simulink model "Boeing787_NewMission_ElectricalThermal_2013"  (R2013a)
settings: Solver=ode23tb  SolverMode=SingleTasking  StartTime=0.0  StopTime=18000  RelTol=1e-3
InitFcn:
  | load('SampleOutput.mat')
  | 
  | load('SampleFuelBurn.mat')
StartFcn:
  | tic
StopFcn:
  | ttt = toc
  | tend = eval(get_param(bdroot,'StopTime'));
  | disp(['Total Simulation Time (s) = ' num2str(ttt) 's']);
  | RTR =  ttt/tend
  | disp(['Simulation Speed is ' num2str(tend/ttt) 'x faster than real-time']);
values from neighbouring files (symbols this model uses):
  CurrentMission = Mission(i)    [mission_plan.m]
  seed = 1    [mission_plan.m]
undefined symbols (not defined in the file or in its folder): FuelBurn
libraries: PowerFlowLib x17, simulink x12, powerlib_meascontrol x1
(part 13 of 17)

== system Boeing787_NewMission_ElectricalThermal_2013/Electrical/230 Vac Distr ==
  note: Generator Bus 1
  note: Generator Bus 2
  Gen 1 : Inport
  Gen 2 : Inport  Port=2
  Gen 3 : Inport  Port=3
  Gen 4 : Inport  Port=4
  Gen 5 : Inport  Port=5
  Gen 6 : Inport  Port=6
  I_Bus : Inport  Port=7
  Gain : Gain  Gain=0.45
  Gain1 : Gain  Gain=0.55
  Gen Bus w/ APU switch : PowerFlowLib/Energy & Power Systems/Electrical/Systems/Gen Bus w// APU switch  LOWVLIMIT=90  UPVLIMIT=250  bus_st=2
  Gen Bus w/ APU switch1 : PowerFlowLib/Energy & Power Systems/Electrical/Systems/Gen Bus w// APU switch  LOWVLIMIT=90  UPVLIMIT=250  bus_st=2
  Terminator : Terminator
  Terminator1 : Terminator
  Vbus1 : Outport
  Vbus2 : Outport  Port=2
  tag scope: i_APU1=global, i_APU2=global, i_GND1=global, i_GND2=global, i_MAIN1=global, i_MAIN2=global
  wires:
  Gen Bus w/ APU switch/3 -> [i_APU1]
  Gen Bus w/ APU switch/4 -> [i_GND1]
  [Gen_Bus1] -> Gen Bus w/ APU switch/1
  Gen Bus w/ APU switch/2 -> [i_MAIN1]
  Gen Bus w/ APU switch1/3 -> [i_APU2]
  Gen Bus w/ APU switch1/4 -> [i_GND2]
  Gen Bus w/ APU switch1/2 -> [i_MAIN2]
  [Gen_Bus2] -> Gen Bus w/ APU switch1/1
  Gen 1/1 -> Gen Bus w/ APU switch/2
  Gen 3/1 -> Gen Bus w/ APU switch1/2
  Gen 5/1 -> Gen Bus w/ APU switch/3
  Gen 6/1 -> Gen Bus w/ APU switch1/3
  Gen Bus w/ APU switch/1 -> Vbus1/1
  Gen Bus w/ APU switch1/1 -> Vbus2/1
  I_Bus/1 -> Gain1/1, Gain/1
  Gain/1 -> Gen Bus w/ APU switch/6
  Gen 2/1 -> Terminator/1
  Gen 4/1 -> Terminator1/1
  Gain1/1 -> Gen Bus w/ APU switch1/6

== system Boeing787_NewMission_ElectricalThermal_2013/Electrical/Auto Transformer ==
  vqd0 : Inport
  iAC : Inport  Port=2
  Constant : Constant
  Constant1 : Constant  Value=115
  Control : Subsystem
  Saturation : Saturate  UpperLimit=20  LowerLimit=0
  Sum1 : Sum  Inputs=|++
  Transformer1 : Subsystem  AncestorBlock=PowerFlowLib/Energy & Power Systems/Electrical/Machines/Transformer  mask(Transformer){Rp=0.005, Rs=0.1, N1=400, N2=200}
      mask prompts: Rp "Primary Winding Resistance"; Rs "Secondary Winding Resistance"; N1 "Number of Turns in Primary"; N2 "Number of Turns in Secondary"
      mask help:
      | The user inputs and outputs are given below. Inputs to the model are:
      |
      | Block Inputs
      | #1: Primary voltage input [V]
      | #2: Secondary current input [A]
      |
      | Block Outputs
      | #1: Secondary voltage output [V]
      | #2: Primary current input [A]
      mask Help: eval('open(''Transformer Help.html'')');
      mask Display:
      | image(imread('Transformer.png'))
      | 
      | port_label('input',1,'{\bf V_i_n}','TexMode','on')
      | port_label('input',2,'{\bf I_o_u_t}','TexMode','on')
      | port_label('input',3,'{\bf u}','TexMode','on')
      | 
      | port_label('output',1,'{\bf V_o_u_t}','TexMode','on')
      | port_label('output',2,'{\bf I_i_n}','TexMode','on')
  vout : Outport
  iqd0 : Outport  Port=2
  wires:
  vqd0/1 -> Transformer1/1(Vin)
  Transformer1/2(Iin) -> iqd0/1
  iAC/1 -> Transformer1/2(Iout)
  Transformer1/1(Vout) -> Control/1(Vout), vout/1
  Sum1/1 -> Saturation/1
  Constant/1 -> Sum1/1
  Constant1/1 -> Control/2(ref)
  Saturation/1 -> Transformer1/3(u)
  Control/1(u) -> Sum1/2

== system Boeing787_NewMission_ElectricalThermal_2013/Electrical/Bus Controls ==
  Constant{1..5} (5 alike) : Constant
  Gen_Bus1 : Outport
  Gen_Bus2 : Outport  Port=2
  270V_DC_Bus : Outport  Port=3
  115V_AC_Bus : Outport  Port=4
  28V_DC_Bus : Outport  Port=5
  wires:
  Constant3/1 -> 28V_DC_Bus/1
  Constant5/1 -> 115V_AC_Bus/1
  Constant2/1 -> 270V_DC_Bus/1
  Constant4/1 -> Gen_Bus2/1
  Constant1/1 -> Gen_Bus1/1

== system Boeing787_NewMission_ElectricalThermal_2013/Electrical/DC Bus 1 ==
  Select : Inport
  VDC_1 : Inport  Port=2
  VDC_2 : Inport  Port=3
  Load current : Inport  Port=4
  Compare To Constant : simulink/Logic and Bit Operations/Compare To Constant  relop=<=  const=3.0  OutDataTypeStr=boolean
  Compare To Constant1 : simulink/Logic and Bit Operations/Compare To Constant  relop=<=  const=3.0  OutDataTypeStr=boolean
  Constant : Constant  Value=[0]
  Multiport Switch : MultiPortSwitch  Inputs=2
  Sum of Elements1 : Sum  Inputs=+
  Switch : Switch  Criteria=u2 ~= 0
  Switch1 : Switch  Criteria=u2 ~= 0
  Vbus : Outport
  IDC_1 : Outport  Port=2
  IDC_2 : Outport  Port=3
  wires:
  Load current/1 -> Sum of Elements1/1
  Multiport Switch/1 -> Vbus/1
  VDC_1/1 -> Multiport Switch/2
  VDC_2/1 -> Multiport Switch/3
  Select/1 -> Multiport Switch/1, Compare To Constant/1, Compare To Constant1/1
  Compare To Constant/1 -> Switch/2
  Compare To Constant1/1 -> Switch1/2
  Constant/1 -> Switch/3, Switch1/3
  Switch/1 -> IDC_1/1
  Switch1/1 -> IDC_2/1
  Sum of Elements1/1 -> Switch1/1, Switch/1

== system Boeing787_NewMission_ElectricalThermal_2013/Electrical/DC Bus 3 ==
  Select : Inport
  VDC_1 : Inport  Port=2
  VDC_2 : Inport  Port=3
  Load current : Inport  Port=4
  Compare To Constant : simulink/Logic and Bit Operations/Compare To Constant  relop=<=  const=3.0  OutDataTypeStr=boolean
  Compare To Constant1 : simulink/Logic and Bit Operations/Compare To Constant  relop=<=  const=3.0  OutDataTypeStr=boolean
  Constant : Constant  Value=[0]
  Multiport Switch : MultiPortSwitch  Inputs=2
  Sum of Elements : Sum  Inputs=+
  Switch : Switch  Criteria=u2 ~= 0
  Switch1 : Switch  Criteria=u2 ~= 0
  Vbus : Outport
  IDC_1 : Outport  Port=2
  IDC_2 : Outport  Port=3
  wires:
  Load current/1 -> Sum of Elements/1
  Multiport Switch/1 -> Vbus/1
  VDC_1/1 -> Multiport Switch/2
  VDC_2/1 -> Multiport Switch/3
  Select/1 -> Multiport Switch/1, Compare To Constant1/1, Compare To Constant/1
  Compare To Constant/1 -> Switch/2
  Compare To Constant1/1 -> Switch1/2
  Constant/1 -> Switch/3, Switch1/3
  Switch/1 -> IDC_1/1
  Switch1/1 -> IDC_2/1
  Sum of Elements/1 -> Switch1/1, Switch/1

== system Boeing787_NewMission_ElectricalThermal_2013/Electrical/Enabled DC Load1 ==
  VDC : Inport
  Control : Inport  Port=2
  Enable : EnablePort
  Demux : Demux  Outputs=2
  Fcn1 : Fcn  Expr=u(1)/(u(2)+0.01)
  Mux : Mux  Inputs=2
  Sum : Sum
  Transfer Fcn : TransferFcn  Denominator=[.01 1]
  iDC : Outport
  wires:
  Control/1 -> Demux/1
  Demux/1 -> Sum/1
  Sum/1 -> Transfer Fcn/1
  VDC/1 -> Mux/2
  Fcn1/1 -> Sum/2
  Mux/1 -> Fcn1/1
  Demux/2 -> Mux/1
  Transfer Fcn/1 -> iDC/1

== system Boeing787_NewMission_ElectricalThermal_2013/Electrical/Enabled_AC_Loadloss ==
  Load Master Vector : Inport
  Vdq0 : Inport  Port=2
  Enable : EnablePort
  Enabled Subsystem : Subsystem  TreatAsAtomicUnit=on
  Enabled Subsystem1 : Subsystem  TreatAsAtomicUnit=on
  Sum1 : Sum  Inputs=|++
  Idq0 : Outport
  loss : Outport  Port=2
  wires:
  Enabled Subsystem/2(loss) -> loss/1
  Load Master Vector/1 -> Enabled Subsystem1/2(Ext vector)
  Sum1/1 -> Idq0/1
  Enabled Subsystem/1(Idq0) -> Sum1/2
  Enabled Subsystem1/1(Idq0) -> Sum1/1
  Vdq0/1 -> Enabled Subsystem/1("Vdq0 "), Enabled Subsystem1/1("Vdq0 ")

== system Boeing787_NewMission_ElectricalThermal_2013/Electrical/Enabled_AC_Loadloss1 ==
  Load Master Vector : Inport
  Vdq0 : Inport  Port=2
  Enable : EnablePort
  Enabled Subsystem : Subsystem  TreatAsAtomicUnit=on
  Enabled Subsystem1 : Subsystem  TreatAsAtomicUnit=on
  Sum1 : Sum  Inputs=|++
  Idq0 : Outport
  loss : Outport  Port=2
  wires:
  Enabled Subsystem/2(loss) -> loss/1
  Load Master Vector/1 -> Enabled Subsystem1/2(Ext vector)
  Sum1/1 -> Idq0/1
  Enabled Subsystem/1(Idq0) -> Sum1/2
  Enabled Subsystem1/1(Idq0) -> Sum1/1
  Vdq0/1 -> Enabled Subsystem1/1("Vdq0 "), Enabled Subsystem/1("Vdq0 ")

== system Boeing787_NewMission_ElectricalThermal_2013/Electrical/Generation Unit Sync-Sync ==
  engine speed : Inport
  battery voltage : Inport  Port=2
  idq0 : Inport  Port=3
  Temperature : Inport  Port=4
  Bus Creator : BusCreator  Inputs=3
  Bus Creator1 : BusCreator  Inputs=3
  Chopper (Averaged) : Subsystem  mask(Chopper.){}
      mask help: Basic chopper. Lossless storage elements. Switching model.
  Coeff of Resistance : Gain  Gain=3.85e-3
  Demux : Demux  Outputs=3
  Dot Product : DotProduct  InputSameDT=on  OutDataTypeStr=Inherit: Inherit via internal rule
  Exciter : Subsystem
      mask Display:
      | p = 0:0.1:(2*pi+0.1);
      | plot(sin(p), cos(p));
      | p1 = (-pi/8-0.1-0.2):0.1:(pi/8+0.1-0.2);
      | plot(0.8*sin(p1), 0.8*cos(p1), 0.8*sin(p1+pi), 0.8*cos(p1+pi));
      | p2 = sin((-pi/8-0.1-0.2+pi/8+0.1-0.2)/2);
      | p3 = sin((-pi/8-0.1-0.2+pi/8+0.1-0.2)/2+pi);
      | p4 = cos((-pi/8-0.1-0.2+pi/8+0.1-0.2)/2);
      | p5 = cos((-pi/8-0.1-0.2+pi/8+0.1-0.2)/2+pi);
      | plot(0.8*[p2, p3], 0.8*[p4, p5]);
      | port_label('output', 1, 'Vdq0');
      | port_label('output', 2, 'Te');
      | port_label('output', 3, 'Vfd');
      | port_label('output', 4, 'Ploss');
      | port_label('input', 1, 'idq0');
      | port_label('input', 2, 'w');
      | port_label('input', 3, 'ifd');
  Gain : Gain  Gain=200*2/3
  Gain1 : Gain  Gain=200
  Gain4 : Gain  Gain=0.001
  Gain5 : Gain  Gain=30
  Gain6 : Gain  Gain=0.02
  Generator : Subsystem
      mask Display:
      | p = 0:0.1:(2*pi+0.1);
      | plot(sin(p), cos(p));
      | p1 = (-pi/8-0.1-0.2):0.1:(pi/8+0.1-0.2);
      | plot(0.8*sin(p1), 0.8*cos(p1), 0.8*sin(p1+pi), 0.8*cos(p1+pi));
      | p2 = sin((-pi/8-0.1-0.2+pi/8+0.1-0.2)/2);
      | p3 = sin((-pi/8-0.1-0.2+pi/8+0.1-0.2)/2+pi);
      | p4 = cos((-pi/8-0.1-0.2+pi/8+0.1-0.2)/2);
      | p5 = cos((-pi/8-0.1-0.2+pi/8+0.1-0.2)/2+pi);
      | plot(0.8*[p2, p3], 0.8*[p4, p5]);
      | port_label('output', 1, 'Vdq0');
      | port_label('output', 2, 'Te');
      | port_label('output', 3, 'Vfd');
      | port_label('output', 4, 'Ploss');
      | port_label('input', 1, 'idq0');
      | port_label('input', 2, 'w');
      | port_label('input', 3, 'ifd');
  Initial Temperature : Constant  Value=25
  Integrator : Integrator  LimitOutput=on  UpperSaturationLimit=10  LowerSaturationLimit=-10
  Integrator1 : Integrator  LimitOutput=on  UpperSaturationLimit=1  LowerSaturationLimit=0
  RPM_to_radps : Gain  Gain=pi/30
  Sqrt : Sqrt  SaturateOnIntegerOverflow=on
  Sum : Sum  Inputs=++|
  Sum1 : Sum
  Sum2 : Sum  Inputs=+-|
  Sum3 : Sum  Inputs=-+|
  Sum4 : Sum  Inputs=+
  Sum5 : Sum  Inputs=|+-
  Sum6 : Sum  Inputs=|++
  Vcmd : Constant  Value=Vnom
  control1 : Constant
  data_sink : PowerFlowLib/Support Functions//Tools/data_sink
  one : Constant
  three-phase active rectifier Voltage Mode : PowerFlowLib/Energy & Power Systems/Electrical/Rectifiers/three-phase  active rectifier Voltage Mode  L=1  C=1e-4
  vdq0 : Outport
  battery current : Outport  Port=2
  engine torque : Outport  Port=3
  Ploss : Outport  Port=4
  wires:
  [R_temp_delta] -> Generator/4(Temp)
  [R_temp_delta] -> Exciter/4(Temp)
  [R_temp_delta] -> Chopper (Averaged)/3(Temperature)
  Sum6/1 -> [R_temp_delta]
  one/1 -> Sum6/2
  Coeff of Resistance/1 -> Sum6/1
  Sum5/1 -> Coeff of Resistance/1
  Initial Temperature/1 -> Sum5/2
  Temperature/1 -> Sum5/1
  engine speed/1 -> RPM_to_radps/1
  Bus Creator1/1 -> Bus Creator/1  "vdq0 (V)"
  Demux/3 -> Bus Creator1/3  "v0"
  Demux/2 -> Bus Creator1/2  "vq"
  Demux/1 -> Bus Creator1/1  "vd"
  Bus Creator/1 -> data_sink/1
  Sum/1 -> engine torque/1
  RPM_to_radps/1 -> Exciter/2(w), Generator/2(w)
  Exciter/1(vdq0) -> three-phase active rectifier Voltage Mode/1
  control1/1 -> three-phase active rectifier Voltage Mode/2
  Generator/3(vfd') -> Gain1/1
  Gain1/1 -> three-phase active rectifier Voltage Mode/3
  Gain/1 -> Bus Creator/3, Generator/3(ifd')  "Exciter current (A)"
  three-phase active rectifier Voltage Mode/1 -> Gain/1
  Exciter/2(Te) -> Sum/1
  Generator/2(Te) -> Sum/2
  idq0/1 -> Generator/1(idq0)
  Generator/1(vdq0) -> Demux/1, vdq0/1, Dot Product/2, Dot Product/1  "Vdq0 (V)"
  Chopper (Averaged)/1(iout) -> Exciter/3(ifd')
  battery voltage/1 -> Chopper (Averaged)/1(vin)
  Chopper (Averaged)/2(iin) -> battery current/1
  Exciter/4(Ploss) -> Sum1/1
  Generator/4(Ploss) -> Sum1/2
  Sum1/1 -> Ploss/1, Bus Creator/2  "Ploss (W)"
  Gain4/1 -> Integrator/1
  Sum2/1 -> Gain4/1
  Integrator/1 -> Sum3/2
  Sum3/1 -> Gain6/1
  Vcmd/1 -> Sum2/1
  Dot Product/1 -> Sum4/1
  Sum4/1 -> Sqrt/1
  Sqrt/1 -> Sum2/2
  Gain6/1 -> Integrator1/1
  Gain5/1 -> Sum3/1
  three-phase active rectifier Voltage Mode/2 -> Exciter/1(idq0)
  Integrator1/1 -> Chopper (Averaged)/2(q), Gain5/1

== system Boeing787_NewMission_ElectricalThermal_2013/Electrical/Generation Unit Sync-Sync1 ==
  engine speed : Inport
  battery voltage : Inport  Port=2
  idq0 : Inport  Port=3
  Temperature : Inport  Port=4
  Bus Creator : BusCreator  Inputs=3
  Bus Creator1 : BusCreator  Inputs=3
  Chopper (Averaged) : Subsystem  mask(Chopper.){}
      mask help: Basic chopper. Lossless storage elements. Switching model.
  Coeff of Resistance : Gain  Gain=3.85e-3
  Demux : Demux  Outputs=3
  Dot Product : DotProduct  InputSameDT=on  OutDataTypeStr=Inherit: Inherit via internal rule
  Exciter : Subsystem
      mask Display:
      | p = 0:0.1:(2*pi+0.1);
      | plot(sin(p), cos(p));
      | p1 = (-pi/8-0.1-0.2):0.1:(pi/8+0.1-0.2);
      | plot(0.8*sin(p1), 0.8*cos(p1), 0.8*sin(p1+pi), 0.8*cos(p1+pi));
      | p2 = sin((-pi/8-0.1-0.2+pi/8+0.1-0.2)/2);
      | p3 = sin((-pi/8-0.1-0.2+pi/8+0.1-0.2)/2+pi);
      | p4 = cos((-pi/8-0.1-0.2+pi/8+0.1-0.2)/2);
      | p5 = cos((-pi/8-0.1-0.2+pi/8+0.1-0.2)/2+pi);
      | plot(0.8*[p2, p3], 0.8*[p4, p5]);
      | port_label('output', 1, 'Vdq0');
      | port_label('output', 2, 'Te');
      | port_label('output', 3, 'Vfd');
      | port_label('output', 4, 'Ploss');
      | port_label('input', 1, 'idq0');
      | port_label('input', 2, 'w');
      | port_label('input', 3, 'ifd');
  Gain : Gain  Gain=200*2/3
  Gain1 : Gain  Gain=200
  Gain4 : Gain  Gain=0.001
  Gain5 : Gain  Gain=30
  Gain6 : Gain  Gain=0.02
  Generator : Subsystem
      mask Display:
      | p = 0:0.1:(2*pi+0.1);
      | plot(sin(p), cos(p));
      | p1 = (-pi/8-0.1-0.2):0.1:(pi/8+0.1-0.2);
      | plot(0.8*sin(p1), 0.8*cos(p1), 0.8*sin(p1+pi), 0.8*cos(p1+pi));
      | p2 = sin((-pi/8-0.1-0.2+pi/8+0.1-0.2)/2);
      | p3 = sin((-pi/8-0.1-0.2+pi/8+0.1-0.2)/2+pi);
      | p4 = cos((-pi/8-0.1-0.2+pi/8+0.1-0.2)/2);
      | p5 = cos((-pi/8-0.1-0.2+pi/8+0.1-0.2)/2+pi);
      | plot(0.8*[p2, p3], 0.8*[p4, p5]);
      | port_label('output', 1, 'Vdq0');
      | port_label('output', 2, 'Te');
      | port_label('output', 3, 'Vfd');
      | port_label('output', 4, 'Ploss');
      | port_label('input', 1, 'idq0');
      | port_label('input', 2, 'w');
      | port_label('input', 3, 'ifd');
  Initial Temperature : Constant  Value=25
  Integrator : Integrator  LimitOutput=on  UpperSaturationLimit=10  LowerSaturationLimit=-10
  Integrator1 : Integrator  LimitOutput=on  UpperSaturationLimit=1  LowerSaturationLimit=0
  RPM_to_radps : Gain  Gain=pi/30
  Sqrt : Sqrt  SaturateOnIntegerOverflow=on
  Sum : Sum  Inputs=++|
  Sum1 : Sum
  Sum2 : Sum  Inputs=+-|
  Sum3 : Sum  Inputs=-+|
  Sum4 : Sum  Inputs=+
  Sum5 : Sum  Inputs=|+-
  Sum6 : Sum  Inputs=|++
  Vcmd : Constant  Value=Vnom
  control1 : Constant
  data_sink : PowerFlowLib/Support Functions//Tools/data_sink
  one : Constant
  three-phase active rectifier Voltage Mode : PowerFlowLib/Energy & Power Systems/Electrical/Rectifiers/three-phase  active rectifier Voltage Mode  L=1  C=1e-4
  vdq0 : Outport
  battery current : Outport  Port=2
  engine torque : Outport  Port=3
  Ploss : Outport  Port=4
  wires:
  Integrator1/1 -> Gain5/1, Chopper (Averaged)/2(q)
  three-phase active rectifier Voltage Mode/2 -> Exciter/1(idq0)
  Gain5/1 -> Sum3/1
  Gain6/1 -> Integrator1/1
  Sqrt/1 -> Sum2/2
  Sum4/1 -> Sqrt/1
  Dot Product/1 -> Sum4/1
  Vcmd/1 -> Sum2/1
  Sum3/1 -> Gain6/1
  Integrator/1 -> Sum3/2
  Sum2/1 -> Gain4/1
  Gain4/1 -> Integrator/1
  Sum1/1 -> Bus Creator/2, Ploss/1  "Ploss (W)"
  Generator/4(Ploss) -> Sum1/2
  Exciter/4(Ploss) -> Sum1/1
  Chopper (Averaged)/2(iin) -> battery current/1
  battery voltage/1 -> Chopper (Averaged)/1(vin)
  Chopper (Averaged)/1(iout) -> Exciter/3(ifd')
  idq0/1 -> Generator/1(idq0)
  Generator/2(Te) -> Sum/2
  Exciter/2(Te) -> Sum/1
  three-phase active rectifier Voltage Mode/1 -> Gain/1
  Gain/1 -> Generator/3(ifd'), Bus Creator/3  "Exciter current (A)"
  Gain1/1 -> three-phase active rectifier Voltage Mode/3
  Generator/3(vfd') -> Gain1/1
  control1/1 -> three-phase active rectifier Voltage Mode/2
  Exciter/1(vdq0) -> three-phase active rectifier Voltage Mode/1
  RPM_to_radps/1 -> Generator/2(w), Exciter/2(w)
  Sum/1 -> engine torque/1
  Bus Creator/1 -> data_sink/1
  Demux/1 -> Bus Creator1/1  "vd"
  Demux/2 -> Bus Creator1/2  "vq"
  Demux/3 -> Bus Creator1/3  "v0"
  Bus Creator1/1 -> Bus Creator/1  "vdq0 (V)"
  engine speed/1 -> RPM_to_radps/1
  Temperature/1 -> Sum5/1
  Initial Temperature/1 -> Sum5/2
  Sum5/1 -> Coeff of Resistance/1
  Coeff of Resistance/1 -> Sum6/1
  one/1 -> Sum6/2
  Sum6/1 -> [R_temp_delta]
  [R_temp_delta] -> Chopper (Averaged)/3(Temperature)
  [R_temp_delta] -> Exciter/4(Temp)
  [R_temp_delta] -> Generator/4(Temp)
  Generator/1(vdq0) -> Dot Product/1, Dot Product/2, vdq0/1, Demux/1  "Vdq0 (V)"

== system Boeing787_NewMission_ElectricalThermal_2013/Electrical/Generation Unit Sync-Sync2 ==
  engine speed : Inport
  battery voltage : Inport  Port=2
  idq0 : Inport  Port=3
  Temperature : Inport  Port=4
  Bus Creator : BusCreator  Inputs=3
  Bus Creator1 : BusCreator  Inputs=3
  Chopper (Averaged) : Subsystem  mask(Chopper.){}
      mask help: Basic chopper. Lossless storage elements. Switching model.
  Coeff of Resistance : Gain  Gain=3.85e-3
  Demux : Demux  Outputs=3
  Dot Product : DotProduct  InputSameDT=on  OutDataTypeStr=Inherit: Inherit via internal rule
  Exciter : Subsystem
      mask Display:
      | p = 0:0.1:(2*pi+0.1);
      | plot(sin(p), cos(p));
      | p1 = (-pi/8-0.1-0.2):0.1:(pi/8+0.1-0.2);
      | plot(0.8*sin(p1), 0.8*cos(p1), 0.8*sin(p1+pi), 0.8*cos(p1+pi));
      | p2 = sin((-pi/8-0.1-0.2+pi/8+0.1-0.2)/2);
      | p3 = sin((-pi/8-0.1-0.2+pi/8+0.1-0.2)/2+pi);
      | p4 = cos((-pi/8-0.1-0.2+pi/8+0.1-0.2)/2);
      | p5 = cos((-pi/8-0.1-0.2+pi/8+0.1-0.2)/2+pi);
      | plot(0.8*[p2, p3], 0.8*[p4, p5]);
      | port_label('output', 1, 'Vdq0');
      | port_label('output', 2, 'Te');
      | port_label('output', 3, 'Vfd');
      | port_label('output', 4, 'Ploss');
      | port_label('input', 1, 'idq0');
      | port_label('input', 2, 'w');
      | port_label('input', 3, 'ifd');
  Gain : Gain  Gain=200*2/3
  Gain1 : Gain  Gain=200
  Gain4 : Gain  Gain=0.001
  Gain5 : Gain  Gain=30
  Gain6 : Gain  Gain=0.02
  Generator : Subsystem
      mask Display:
      | p = 0:0.1:(2*pi+0.1);
      | plot(sin(p), cos(p));
      | p1 = (-pi/8-0.1-0.2):0.1:(pi/8+0.1-0.2);
      | plot(0.8*sin(p1), 0.8*cos(p1), 0.8*sin(p1+pi), 0.8*cos(p1+pi));
      | p2 = sin((-pi/8-0.1-0.2+pi/8+0.1-0.2)/2);
      | p3 = sin((-pi/8-0.1-0.2+pi/8+0.1-0.2)/2+pi);
      | p4 = cos((-pi/8-0.1-0.2+pi/8+0.1-0.2)/2);
      | p5 = cos((-pi/8-0.1-0.2+pi/8+0.1-0.2)/2+pi);
      | plot(0.8*[p2, p3], 0.8*[p4, p5]);
      | port_label('output', 1, 'Vdq0');
      | port_label('output', 2, 'Te');
      | port_label('output', 3, 'Vfd');
      | port_label('output', 4, 'Ploss');
      | port_label('input', 1, 'idq0');
      | port_label('input', 2, 'w');
      | port_label('input', 3, 'ifd');
  Initial Temperature : Constant  Value=25
  Integrator : Integrator  LimitOutput=on  UpperSaturationLimit=10  LowerSaturationLimit=-10
  Integrator1 : Integrator  LimitOutput=on  UpperSaturationLimit=1  LowerSaturationLimit=0
  RPM_to_radps : Gain  Gain=pi/30
  Sqrt : Sqrt  SaturateOnIntegerOverflow=on
  Sum : Sum  Inputs=++|
  Sum1 : Sum
  Sum2 : Sum  Inputs=+-|
  Sum3 : Sum  Inputs=-+|
  Sum4 : Sum  Inputs=+
  Sum5 : Sum  Inputs=|+-
  Sum6 : Sum  Inputs=|++
  Vcmd : Constant  Value=Vnom
  control1 : Constant
  data_sink : PowerFlowLib/Support Functions//Tools/data_sink
  one : Constant
  three-phase active rectifier Voltage Mode : PowerFlowLib/Energy & Power Systems/Electrical/Rectifiers/three-phase  active rectifier Voltage Mode  L=1  C=1e-4
  vdq0 : Outport
  battery current : Outport  Port=2
  engine torque : Outport  Port=3
  Ploss : Outport  Port=4
  wires:
  [R_temp_delta] -> Generator/4(Temp)
  [R_temp_delta] -> Exciter/4(Temp)
  [R_temp_delta] -> Chopper (Averaged)/3(Temperature)
  Sum6/1 -> [R_temp_delta]
  one/1 -> Sum6/2
  Coeff of Resistance/1 -> Sum6/1
  Sum5/1 -> Coeff of Resistance/1
  Initial Temperature/1 -> Sum5/2
  Temperature/1 -> Sum5/1
  engine speed/1 -> RPM_to_radps/1
  Bus Creator1/1 -> Bus Creator/1  "vdq0 (V)"
  Demux/3 -> Bus Creator1/3  "v0"
  Demux/2 -> Bus Creator1/2  "vq"
  Demux/1 -> Bus Creator1/1  "vd"
  Bus Creator/1 -> data_sink/1
  Sum/1 -> engine torque/1
  RPM_to_radps/1 -> Exciter/2(w), Generator/2(w)
  Exciter/1(vdq0) -> three-phase active rectifier Voltage Mode/1
  control1/1 -> three-phase active rectifier Voltage Mode/2
  Generator/3(vfd') -> Gain1/1
  Gain1/1 -> three-phase active rectifier Voltage Mode/3
  Gain/1 -> Bus Creator/3, Generator/3(ifd')  "Exciter current (A)"
  three-phase active rectifier Voltage Mode/1 -> Gain/1
  Exciter/2(Te) -> Sum/1
  Generator/2(Te) -> Sum/2
  idq0/1 -> Generator/1(idq0)
  Generator/1(vdq0) -> Demux/1, vdq0/1, Dot Product/2, Dot Product/1  "Vdq0 (V)"
  Chopper (Averaged)/1(iout) -> Exciter/3(ifd')
  battery voltage/1 -> Chopper (Averaged)/1(vin)
  Chopper (Averaged)/2(iin) -> battery current/1
  Exciter/4(Ploss) -> Sum1/1
  Generator/4(Ploss) -> Sum1/2
  Sum1/1 -> Ploss/1, Bus Creator/2  "Ploss (W)"
  Gain4/1 -> Integrator/1
  Sum2/1 -> Gain4/1
  Integrator/1 -> Sum3/2
  Sum3/1 -> Gain6/1
  Vcmd/1 -> Sum2/1
  Dot Product/1 -> Sum4/1
  Sum4/1 -> Sqrt/1
  Sqrt/1 -> Sum2/2
  Gain6/1 -> Integrator1/1
  Gain5/1 -> Sum3/1
  three-phase active rectifier Voltage Mode/2 -> Exciter/1(idq0)
  Integrator1/1 -> Chopper (Averaged)/2(q), Gain5/1

== system Boeing787_NewMission_ElectricalThermal_2013/Electrical/Generation Unit Sync-Sync3 ==
  engine speed : Inport
  battery voltage : Inport  Port=2
  idq0 : Inport  Port=3
  Temperature : Inport  Port=4
  Bus Creator : BusCreator  Inputs=3
  Bus Creator1 : BusCreator  Inputs=3
  Chopper (Averaged) : Subsystem  mask(Chopper.){}
      mask help: Basic chopper. Lossless storage elements. Switching model.
  Coeff of Resistance : Gain  Gain=3.85e-3
  Demux : Demux  Outputs=3
  Dot Product : DotProduct  InputSameDT=on  OutDataTypeStr=Inherit: Inherit via internal rule
  Exciter : Subsystem
      mask Display:
      | p = 0:0.1:(2*pi+0.1);
      | plot(sin(p), cos(p));
      | p1 = (-pi/8-0.1-0.2):0.1:(pi/8+0.1-0.2);
      | plot(0.8*sin(p1), 0.8*cos(p1), 0.8*sin(p1+pi), 0.8*cos(p1+pi));
      | p2 = sin((-pi/8-0.1-0.2+pi/8+0.1-0.2)/2);
      | p3 = sin((-pi/8-0.1-0.2+pi/8+0.1-0.2)/2+pi);
      | p4 = cos((-pi/8-0.1-0.2+pi/8+0.1-0.2)/2);
      | p5 = cos((-pi/8-0.1-0.2+pi/8+0.1-0.2)/2+pi);
      | plot(0.8*[p2, p3], 0.8*[p4, p5]);
      | port_label('output', 1, 'Vdq0');
      | port_label('output', 2, 'Te');
      | port_label('output', 3, 'Vfd');
      | port_label('output', 4, 'Ploss');
      | port_label('input', 1, 'idq0');
      | port_label('input', 2, 'w');
      | port_label('input', 3, 'ifd');
  Gain : Gain  Gain=200*2/3
  Gain1 : Gain  Gain=200
  Gain4 : Gain  Gain=0.001
  Gain5 : Gain  Gain=30
  Gain6 : Gain  Gain=0.02
  Generator : Subsystem
      mask Display:
      | p = 0:0.1:(2*pi+0.1);
      | plot(sin(p), cos(p));
      | p1 = (-pi/8-0.1-0.2):0.1:(pi/8+0.1-0.2);
      | plot(0.8*sin(p1), 0.8*cos(p1), 0.8*sin(p1+pi), 0.8*cos(p1+pi));
      | p2 = sin((-pi/8-0.1-0.2+pi/8+0.1-0.2)/2);
      | p3 = sin((-pi/8-0.1-0.2+pi/8+0.1-0.2)/2+pi);
      | p4 = cos((-pi/8-0.1-0.2+pi/8+0.1-0.2)/2);
      | p5 = cos((-pi/8-0.1-0.2+pi/8+0.1-0.2)/2+pi);
      | plot(0.8*[p2, p3], 0.8*[p4, p5]);
      | port_label('output', 1, 'Vdq0');
      | port_label('output', 2, 'Te');
      | port_label('output', 3, 'Vfd');
      | port_label('output', 4, 'Ploss');
      | port_label('input', 1, 'idq0');
      | port_label('input', 2, 'w');
      | port_label('input', 3, 'ifd');
  Initial Temperature : Constant  Value=25
  Integrator : Integrator  LimitOutput=on  UpperSaturationLimit=10  LowerSaturationLimit=-10
  Integrator1 : Integrator  LimitOutput=on  UpperSaturationLimit=1  LowerSaturationLimit=0
  RPM_to_radps : Gain  Gain=pi/30
  Sqrt : Sqrt  SaturateOnIntegerOverflow=on
  Sum : Sum  Inputs=++|
  Sum1 : Sum
  Sum2 : Sum  Inputs=+-|
  Sum3 : Sum  Inputs=-+|
  Sum4 : Sum  Inputs=+
  Sum5 : Sum  Inputs=|+-
  Sum6 : Sum  Inputs=|++
  Vcmd : Constant  Value=Vnom
  control1 : Constant
  data_sink : PowerFlowLib/Support Functions//Tools/data_sink
  one : Constant
  three-phase active rectifier Voltage Mode : PowerFlowLib/Energy & Power Systems/Electrical/Rectifiers/three-phase  active rectifier Voltage Mode  L=1  C=1e-4
  vdq0 : Outport
  battery current : Outport  Port=2
  engine torque : Outport  Port=3
  Ploss : Outport  Port=4
  wires:
  Integrator1/1 -> Gain5/1, Chopper (Averaged)/2(q)
  three-phase active rectifier Voltage Mode/2 -> Exciter/1(idq0)
  Gain5/1 -> Sum3/1
  Gain6/1 -> Integrator1/1
  Sqrt/1 -> Sum2/2
  Sum4/1 -> Sqrt/1
  Dot Product/1 -> Sum4/1
  Vcmd/1 -> Sum2/1
  Sum3/1 -> Gain6/1
  Integrator/1 -> Sum3/2
  Sum2/1 -> Gain4/1
  Gain4/1 -> Integrator/1
  Sum1/1 -> Bus Creator/2, Ploss/1  "Ploss (W)"
  Generator/4(Ploss) -> Sum1/2
  Exciter/4(Ploss) -> Sum1/1
  Chopper (Averaged)/2(iin) -> battery current/1
  battery voltage/1 -> Chopper (Averaged)/1(vin)
  Chopper (Averaged)/1(iout) -> Exciter/3(ifd')
  Generator/1(vdq0) -> Dot Product/1, Dot Product/2, vdq0/1, Demux/1  "Vdq0 (V)"
  idq0/1 -> Generator/1(idq0)
  Generator/2(Te) -> Sum/2
  Exciter/2(Te) -> Sum/1
  three-phase active rectifier Voltage Mode/1 -> Gain/1
  Gain/1 -> Generator/3(ifd'), Bus Creator/3  "Exciter current (A)"
  Gain1/1 -> three-phase active rectifier Voltage Mode/3
  Generator/3(vfd') -> Gain1/1
  control1/1 -> three-phase active rectifier Voltage Mode/2
  Exciter/1(vdq0) -> three-phase active rectifier Voltage Mode/1
  RPM_to_radps/1 -> Generator/2(w), Exciter/2(w)
  Sum/1 -> engine torque/1
  Bus Creator/1 -> data_sink/1
  Demux/1 -> Bus Creator1/1  "vd"
  Demux/2 -> Bus Creator1/2  "vq"
  Demux/3 -> Bus Creator1/3  "v0"
  Bus Creator1/1 -> Bus Creator/1  "vdq0 (V)"
  engine speed/1 -> RPM_to_radps/1
  Temperature/1 -> Sum5/1
  Initial Temperature/1 -> Sum5/2
  Sum5/1 -> Coeff of Resistance/1
  Coeff of Resistance/1 -> Sum6/1
  one/1 -> Sum6/2
  Sum6/1 -> [R_temp_delta]
  [R_temp_delta] -> Chopper (Averaged)/3(Temperature)
  [R_temp_delta] -> Exciter/4(Temp)
  [R_temp_delta] -> Generator/4(Temp)

== system Boeing787_NewMission_ElectricalThermal_2013/Electrical/Generation Unit Sync-Sync4 ==
  engine speed : Inport
  battery voltage : Inport  Port=2
  idq0 : Inport  Port=3
  Temperature : Inport  Port=4
  Bus Creator : BusCreator  Inputs=3
  Bus Creator1 : BusCreator  Inputs=3
  Chopper (Averaged) : Subsystem  mask(Chopper.){}
      mask help: Basic chopper. Lossless storage elements. Switching model.
  Coeff of Resistance : Gain  Gain=3.85e-3
  Demux : Demux  Outputs=3
  Dot Product : DotProduct  InputSameDT=on  OutDataTypeStr=Inherit: Inherit via internal rule
  Exciter : Subsystem
      mask Display:
      | p = 0:0.1:(2*pi+0.1);
      | plot(sin(p), cos(p));
      | p1 = (-pi/8-0.1-0.2):0.1:(pi/8+0.1-0.2);
      | plot(0.8*sin(p1), 0.8*cos(p1), 0.8*sin(p1+pi), 0.8*cos(p1+pi));
      | p2 = sin((-pi/8-0.1-0.2+pi/8+0.1-0.2)/2);
      | p3 = sin((-pi/8-0.1-0.2+pi/8+0.1-0.2)/2+pi);
      | p4 = cos((-pi/8-0.1-0.2+pi/8+0.1-0.2)/2);
      | p5 = cos((-pi/8-0.1-0.2+pi/8+0.1-0.2)/2+pi);
      | plot(0.8*[p2, p3], 0.8*[p4, p5]);
      | port_label('output', 1, 'Vdq0');
      | port_label('output', 2, 'Te');
      | port_label('output', 3, 'Vfd');
      | port_label('output', 4, 'Ploss');
      | port_label('input', 1, 'idq0');
      | port_label('input', 2, 'w');
      | port_label('input', 3, 'ifd');
  Gain : Gain  Gain=200*2/3
  Gain1 : Gain  Gain=200
  Gain4 : Gain  Gain=0.001
  Gain5 : Gain  Gain=30
  Gain6 : Gain  Gain=0.02
  Generator : Subsystem
      mask Display:
      | p = 0:0.1:(2*pi+0.1);
      | plot(sin(p), cos(p));
      | p1 = (-pi/8-0.1-0.2):0.1:(pi/8+0.1-0.2);
      | plot(0.8*sin(p1), 0.8*cos(p1), 0.8*sin(p1+pi), 0.8*cos(p1+pi));
      | p2 = sin((-pi/8-0.1-0.2+pi/8+0.1-0.2)/2);
      | p3 = sin((-pi/8-0.1-0.2+pi/8+0.1-0.2)/2+pi);
      | p4 = cos((-pi/8-0.1-0.2+pi/8+0.1-0.2)/2);
      | p5 = cos((-pi/8-0.1-0.2+pi/8+0.1-0.2)/2+pi);
      | plot(0.8*[p2, p3], 0.8*[p4, p5]);
      | port_label('output', 1, 'Vdq0');
      | port_label('output', 2, 'Te');
      | port_label('output', 3, 'Vfd');
      | port_label('output', 4, 'Ploss');
      | port_label('input', 1, 'idq0');
      | port_label('input', 2, 'w');
      | port_label('input', 3, 'ifd');
  Initial Temperature : Constant  Value=25
  Integrator : Integrator  LimitOutput=on  UpperSaturationLimit=10  LowerSaturationLimit=-10
  Integrator1 : Integrator  LimitOutput=on  UpperSaturationLimit=1  LowerSaturationLimit=0
  RPM_to_radps : Gain  Gain=pi/30
  Sqrt : Sqrt  SaturateOnIntegerOverflow=on
  Sum : Sum  Inputs=++|
  Sum1 : Sum
  Sum2 : Sum  Inputs=+-|
  Sum3 : Sum  Inputs=-+|
  Sum4 : Sum  Inputs=+
  Sum5 : Sum  Inputs=|+-
  Sum6 : Sum  Inputs=|++
  Vcmd : Constant  Value=Vnom
  control1 : Constant
  data_sink : PowerFlowLib/Support Functions//Tools/data_sink
  one : Constant
  three-phase active rectifier Voltage Mode : PowerFlowLib/Energy & Power Systems/Electrical/Rectifiers/three-phase  active rectifier Voltage Mode  L=1  C=1e-4
  vdq0 : Outport
  battery current : Outport  Port=2
  engine torque : Outport  Port=3
  Ploss : Outport  Port=4
  wires:
  [R_temp_delta] -> Generator/4(Temp)
  [R_temp_delta] -> Exciter/4(Temp)
  [R_temp_delta] -> Chopper (Averaged)/3(Temperature)
  Sum6/1 -> [R_temp_delta]
  one/1 -> Sum6/2
  Coeff of Resistance/1 -> Sum6/1
  Sum5/1 -> Coeff of Resistance/1
  Initial Temperature/1 -> Sum5/2
  Temperature/1 -> Sum5/1
  engine speed/1 -> RPM_to_radps/1
  Bus Creator1/1 -> Bus Creator/1  "vdq0 (V)"
  Demux/3 -> Bus Creator1/3  "v0"
  Demux/2 -> Bus Creator1/2  "vq"
  Demux/1 -> Bus Creator1/1  "vd"
  Bus Creator/1 -> data_sink/1
  Sum/1 -> engine torque/1
  RPM_to_radps/1 -> Exciter/2(w), Generator/2(w)
  Exciter/1(vdq0) -> three-phase active rectifier Voltage Mode/1
  control1/1 -> three-phase active rectifier Voltage Mode/2
  Generator/3(vfd') -> Gain1/1
  Gain1/1 -> three-phase active rectifier Voltage Mode/3
  Gain/1 -> Bus Creator/3, Generator/3(ifd')  "Exciter current (A)"
  three-phase active rectifier Voltage Mode/1 -> Gain/1
  Exciter/2(Te) -> Sum/1
  Generator/2(Te) -> Sum/2
  idq0/1 -> Generator/1(idq0)
  Generator/1(vdq0) -> Demux/1, vdq0/1, Dot Product/2, Dot Product/1  "Vdq0 (V)"
  Chopper (Averaged)/1(iout) -> Exciter/3(ifd')
  battery voltage/1 -> Chopper (Averaged)/1(vin)
  Chopper (Averaged)/2(iin) -> battery current/1
  Exciter/4(Ploss) -> Sum1/1
  Generator/4(Ploss) -> Sum1/2
  Sum1/1 -> Ploss/1, Bus Creator/2  "Ploss (W)"
  Gain4/1 -> Integrator/1
  Sum2/1 -> Gain4/1
  Integrator/1 -> Sum3/2
  Sum3/1 -> Gain6/1
  Vcmd/1 -> Sum2/1
  Dot Product/1 -> Sum4/1
  Sum4/1 -> Sqrt/1
  Sqrt/1 -> Sum2/2
  Gain6/1 -> Integrator1/1
  Gain5/1 -> Sum3/1
  three-phase active rectifier Voltage Mode/2 -> Exciter/1(idq0)
  Integrator1/1 -> Chopper (Averaged)/2(q), Gain5/1

== system Boeing787_NewMission_ElectricalThermal_2013/Electrical/Generation Unit Sync-Sync5 ==
  engine speed : Inport
  battery voltage : Inport  Port=2
  idq0 : Inport  Port=3
  Temperature : Inport  Port=4
  Bus Creator : BusCreator  Inputs=3
  Bus Creator1 : BusCreator  Inputs=3
  Chopper (Averaged) : Subsystem  mask(Chopper.){}
      mask help: Basic chopper. Lossless storage elements. Switching model.
  Coeff of Resistance : Gain  Gain=3.85e-3
  Demux : Demux  Outputs=3
  Dot Product : DotProduct  InputSameDT=on  OutDataTypeStr=Inherit: Inherit via internal rule
  Exciter : Subsystem
      mask Display:
      | p = 0:0.1:(2*pi+0.1);
      | plot(sin(p), cos(p));
      | p1 = (-pi/8-0.1-0.2):0.1:(pi/8+0.1-0.2);
      | plot(0.8*sin(p1), 0.8*cos(p1), 0.8*sin(p1+pi), 0.8*cos(p1+pi));
      | p2 = sin((-pi/8-0.1-0.2+pi/8+0.1-0.2)/2);
      | p3 = sin((-pi/8-0.1-0.2+pi/8+0.1-0.2)/2+pi);
      | p4 = cos((-pi/8-0.1-0.2+pi/8+0.1-0.2)/2);
      | p5 = cos((-pi/8-0.1-0.2+pi/8+0.1-0.2)/2+pi);
      | plot(0.8*[p2, p3], 0.8*[p4, p5]);
      | port_label('output', 1, 'Vdq0');
      | port_label('output', 2, 'Te');
      | port_label('output', 3, 'Vfd');
      | port_label('output', 4, 'Ploss');
      | port_label('input', 1, 'idq0');
      | port_label('input', 2, 'w');
      | port_label('input', 3, 'ifd');
  Gain : Gain  Gain=200*2/3
  Gain1 : Gain  Gain=200
  Gain4 : Gain  Gain=0.001
  Gain5 : Gain  Gain=30
  Gain6 : Gain  Gain=0.02
  Generator : Subsystem
      mask Display:
      | p = 0:0.1:(2*pi+0.1);
      | plot(sin(p), cos(p));
      | p1 = (-pi/8-0.1-0.2):0.1:(pi/8+0.1-0.2);
      | plot(0.8*sin(p1), 0.8*cos(p1), 0.8*sin(p1+pi), 0.8*cos(p1+pi));
      | p2 = sin((-pi/8-0.1-0.2+pi/8+0.1-0.2)/2);
      | p3 = sin((-pi/8-0.1-0.2+pi/8+0.1-0.2)/2+pi);
      | p4 = cos((-pi/8-0.1-0.2+pi/8+0.1-0.2)/2);
      | p5 = cos((-pi/8-0.1-0.2+pi/8+0.1-0.2)/2+pi);
      | plot(0.8*[p2, p3], 0.8*[p4, p5]);
      | port_label('output', 1, 'Vdq0');
      | port_label('output', 2, 'Te');
      | port_label('output', 3, 'Vfd');
      | port_label('output', 4, 'Ploss');
      | port_label('input', 1, 'idq0');
      | port_label('input', 2, 'w');
      | port_label('input', 3, 'ifd');
  Initial Temperature : Constant  Value=25
  Integrator : Integrator  LimitOutput=on  UpperSaturationLimit=10  LowerSaturationLimit=-10
  Integrator1 : Integrator  LimitOutput=on  UpperSaturationLimit=1  LowerSaturationLimit=0
  RPM_to_radps : Gain  Gain=pi/30
  Sqrt : Sqrt  SaturateOnIntegerOverflow=on
  Sum : Sum  Inputs=++|
  Sum1 : Sum
  Sum2 : Sum  Inputs=+-|
  Sum3 : Sum  Inputs=-+|
  Sum4 : Sum  Inputs=+
  Sum5 : Sum  Inputs=|+-
  Sum6 : Sum  Inputs=|++
  Vcmd : Constant  Value=Vnom
  control1 : Constant
  data_sink : PowerFlowLib/Support Functions//Tools/data_sink
  one : Constant
  three-phase active rectifier Voltage Mode : PowerFlowLib/Energy & Power Systems/Electrical/Rectifiers/three-phase  active rectifier Voltage Mode  L=1  C=1e-4
  vdq0 : Outport
  battery current : Outport  Port=2
  engine torque : Outport  Port=3
  Ploss : Outport  Port=4
  wires:
  Integrator1/1 -> Gain5/1, Chopper (Averaged)/2(q)
  three-phase active rectifier Voltage Mode/2 -> Exciter/1(idq0)
  Gain5/1 -> Sum3/1
  Gain6/1 -> Integrator1/1
  Sqrt/1 -> Sum2/2
  Sum4/1 -> Sqrt/1
  Dot Product/1 -> Sum4/1
  Vcmd/1 -> Sum2/1
  Sum3/1 -> Gain6/1
  Integrator/1 -> Sum3/2
  Sum2/1 -> Gain4/1
  Gain4/1 -> Integrator/1
  Sum1/1 -> Bus Creator/2, Ploss/1  "Ploss (W)"
  Generator/4(Ploss) -> Sum1/2
  Exciter/4(Ploss) -> Sum1/1
  Chopper (Averaged)/2(iin) -> battery current/1
  battery voltage/1 -> Chopper (Averaged)/1(vin)
  Chopper (Averaged)/1(iout) -> Exciter/3(ifd')
  Generator/1(vdq0) -> Dot Product/1, Dot Product/2, vdq0/1, Demux/1  "Vdq0 (V)"
  idq0/1 -> Generator/1(idq0)
  Generator/2(Te) -> Sum/2
  Exciter/2(Te) -> Sum/1
  three-phase active rectifier Voltage Mode/1 -> Gain/1
  Gain/1 -> Generator/3(ifd'), Bus Creator/3  "Exciter current (A)"
  Gain1/1 -> three-phase active rectifier Voltage Mode/3
  Generator/3(vfd') -> Gain1/1
  control1/1 -> three-phase active rectifier Voltage Mode/2
  Exciter/1(vdq0) -> three-phase active rectifier Voltage Mode/1
  RPM_to_radps/1 -> Generator/2(w), Exciter/2(w)
  Sum/1 -> engine torque/1
  Bus Creator/1 -> data_sink/1
  Demux/1 -> Bus Creator1/1  "vd"
  Demux/2 -> Bus Creator1/2  "vq"
  Demux/3 -> Bus Creator1/3  "v0"
  Bus Creator1/1 -> Bus Creator/1  "vdq0 (V)"
  engine speed/1 -> RPM_to_radps/1
  Temperature/1 -> Sum5/1
  Initial Temperature/1 -> Sum5/2
  Sum5/1 -> Coeff of Resistance/1
  Coeff of Resistance/1 -> Sum6/1
  one/1 -> Sum6/2
  Sum6/1 -> [R_temp_delta]
  [R_temp_delta] -> Chopper (Averaged)/3(Temperature)
  [R_temp_delta] -> Exciter/4(Temp)
  [R_temp_delta] -> Generator/4(Temp)

== system Boeing787_NewMission_ElectricalThermal_2013/Electrical/Loads ==
  115VAC : Lookup_n-D  NumberOfTableDimensions=1  BreakpointsForDimension1=CurrentMission.tvec  Table=CurrentMission.V115ac  InterpMethod=Flat  RndMeth=Simplest  InputSameDT=on
  230VAC : Lookup_n-D  NumberOfTableDimensions=1  BreakpointsForDimension1=CurrentMission.tvec  Table=CurrentMission.V230ac  InterpMethod=Flat  RndMeth=Simplest  InputSameDT=on
  270VDC : Lookup_n-D  NumberOfTableDimensions=1  BreakpointsForDimension1=CurrentMission.tvec  Table=CurrentMission.V270dc  InterpMethod=Flat  RndMeth=Simplest  InputSameDT=on
  28VDC : Lookup_n-D  NumberOfTableDimensions=1  BreakpointsForDimension1=CurrentMission.tvec  Table=CurrentMission.V28dc  InterpMethod=Flat  RndMeth=Simplest  InputSameDT=on
  Clock : Clock
  Constant{,1..3} (4 alike) : Constant  Value=0
  Mux{,1..3} (4 alike) : Mux  Inputs=3
  PF1 : Gain  Gain=0
  PF2 : Gain  Gain=0.329
  PF3 : Gain  Gain=0.329
  PF4 : Gain  Gain=0
  Product{,1..3} (4 alike) : Product
  Uniform Random Number : UniformRandomNumber  Minimum=0.95  Maximum=1.05  Seed=seed+500  SampleTime=1
  Uniform Random Number1 : UniformRandomNumber  Minimum=0.95  Maximum=1.05  Seed=seed  SampleTime=1
  Uniform Random Number2 : UniformRandomNumber  Minimum=0.95  Maximum=1.05  SampleTime=1
  Uniform Random Number3 : UniformRandomNumber  Minimum=0.95  Maximum=1.05  SampleTime=1
  kW to W : Gain  Gain=1000
  kW to W1 : Gain  Gain=1000
  kW to W2 : Gain  Gain=1000
  kW to W3 : Gain  Gain=0
  230 Vac Loads : Outport
  115 Vac Loads : Outport  Port=2
  270 Vdc Loads : Outport  Port=3
  28 Vdc Loads : Outport  Port=4
  wires:
  Mux2/1 -> 230 Vac Loads/1
  Mux/1 -> 270 Vdc Loads/1
  Clock/1 -> 28VDC/1, 270VDC/1, 115VAC/1, 230VAC/1
  PF3/1 -> Mux/2  "Q"
  270VDC/1 -> kW to W1/1  "P"
  PF2/1 -> Mux1/2  "Q"
  115VAC/1 -> kW to W2/1  "P"
  PF1/1 -> Mux2/2  "Q"
  230VAC/1 -> kW to W/1  "P"
  PF4/1 -> Mux3/2  "Q"
  28VDC/1 -> kW to W3/1  "P"
  Mux3/1 -> 28 Vdc Loads/1
  Constant/1 -> Mux/3
  Constant1/1 -> Mux3/3
  Constant2/1 -> Mux1/3
  Constant3/1 -> Mux2/3
  Mux1/1 -> 115 Vac Loads/1
  Product1/1 -> PF1/1, Mux2/1
  Product/1 -> PF2/1, Mux1/1
  Product2/1 -> PF3/1, Mux/1
  Product3/1 -> PF4/1, Mux3/1
  kW to W2/1 -> Product/2
  kW to W/1 -> Product1/2
  kW to W1/1 -> Product2/2
  Uniform Random Number3/1 -> Product3/1
  Uniform Random Number2/1 -> Product2/1
  kW to W3/1 -> Product3/2

== system Boeing787_NewMission_ElectricalThermal_2013/Electrical/Outputs ==
  Left_Wing_Toqrue_Nm : Inport
  Rght_Wing_Torque_Nm : Inport  Port=2
  APU_Torque_Nm : Inport  Port=3
  DC_Voltage_270 : Inport  Port=4
  Bus Creator : BusCreator  Inputs=4
  Electrical : Outport
  wires:
  Rght_Wing_Torque_Nm/1 -> Bus Creator/2  "Right Wing Torq (Nm)"
  APU_Torque_Nm/1 -> Bus Creator/3  "APU Torq (Nm)"
  Left_Wing_Toqrue_Nm/1 -> Bus Creator/1  "Left Wing Torq (Nm)"
  Bus Creator/1 -> Electrical/1
  DC_Voltage_270/1 -> Bus Creator/4  "DC_Voltage_270"

== system Boeing787_NewMission_ElectricalThermal_2013/Electrical/Thermal Interface ==
  Generator Loss [4] : Inport
  APU Loss [2] : Inport  Port=2
  Battery Loss [1] : Inport  Port=3
  Loadloss_W : Inport  Port=4
  Battery Thermal Model : Subsystem
  Constant{,1,3..4} (4 alike) : Constant  Value=0
  Constant2 : Constant  Value=25
  Constant5 : Constant  Value=25
  Coolant Temp : Constant  Value=25
  Coolant mdot : Constant  Value=0.5
  Demux : Demux
  Demux1 : Demux  Outputs=2
  Gain : Gain  Gain=50
  Generator 1 Thermal Model : Subsystem
  Generator 2 Thermal Model : Subsystem
  Generator 3 Thermal Model : Subsystem
  Generator 4 Thermal Model : Subsystem
  Generator 5 Thermal Model : Subsystem
  Generator 6 Thermal Model : Subsystem
  Load Thermal Model : Subsystem
  Mux : Mux
  To Workspace6 : ToWorkspace  VariableName=gen_temps  SaveFormat=Structure With Time  SampleTime=-1
  air Temp : Constant  Value=25
  Tgen1 : Outport
  Tgen2 : Outport  Port=2
  Tgen3 : Outport  Port=3
  Tgen4 : Outport  Port=4
  Tgen5 : Outport  Port=5
  Tgen6 : Outport  Port=6
  Tbatt : Outport  Port=7
  TLoad : Outport  Port=8
  wires:
  Generator Loss [4]/1 -> Gain/1
  Demux/1 -> Generator 1 Thermal Model/1(Ploss)
  Demux/2 -> Generator 2 Thermal Model/1(Ploss)
  Demux/3 -> Generator 3 Thermal Model/1(Ploss)
  Demux/4 -> Generator 4 Thermal Model/1(Ploss)
  Generator 4 Thermal Model/1(T_gen) -> Mux/4, Tgen4/1
  Generator 2 Thermal Model/1(T_gen) -> Mux/2, Tgen2/1
  Generator 1 Thermal Model/1(T_gen) -> Mux/1, Tgen1/1
  APU Loss [2]/1 -> Demux1/1
  Demux1/1 -> Generator 5 Thermal Model/1(Ploss)
  Demux1/2 -> Generator 6 Thermal Model/1(Ploss)
  Generator 6 Thermal Model/1(T_gen) -> Tgen6/1
  Generator 5 Thermal Model/1(T_gen) -> Tgen5/1
  Coolant Temp/1 -> [Tf]
  air Temp/1 -> [Ta]
  Coolant mdot/1 -> [mdot]
  [mdot] -> Generator 1 Thermal Model/4(coolant mdot)
  [Tf] -> Generator 1 Thermal Model/2(Liquid Coolant Temp)
  [Ta] -> Generator 1 Thermal Model/3(Air Temp)
  [Tf] -> Generator 6 Thermal Model/2(Liquid Coolant Temp)
  [Ta] -> Generator 6 Thermal Model/3(Air Temp)
  [mdot] -> Generator 6 Thermal Model/4(coolant mdot)
  [Tf] -> Generator 5 Thermal Model/2(Liquid Coolant Temp)
  [Ta] -> Generator 5 Thermal Model/3(Air Temp)
  [mdot] -> Generator 5 Thermal Model/4(coolant mdot)
  [mdot] -> Generator 4 Thermal Model/4(coolant mdot)
  [Ta] -> Generator 4 Thermal Model/3(Air Temp)
  [Tf] -> Generator 4 Thermal Model/2(Liquid Coolant Temp)
  [Tf] -> Generator 3 Thermal Model/2(Liquid Coolant Temp)
  [Ta] -> Generator 3 Thermal Model/3(Air Temp)
  [mdot] -> Generator 3 Thermal Model/4(coolant mdot)
  [Tf] -> Generator 2 Thermal Model/2(Liquid Coolant Temp)
  [mdot] -> Generator 2 Thermal Model/4(coolant mdot)
  [Ta] -> Generator 2 Thermal Model/3(Air Temp)
  Battery Loss [1]/1 -> Battery Thermal Model/1(Ploss)
  Loadloss_W/1 -> Load Thermal Model/1(Ploss)
  Constant/1 -> Battery Thermal Model/2(Liquid Coolant Temp)
  Constant1/1 -> Battery Thermal Model/4(coolant mdot)
  Constant2/1 -> Battery Thermal Model/3(Air Temp)
  Constant4/1 -> Load Thermal Model/4(coolant mdot)
  Constant3/1 -> Load Thermal Model/2(Liquid Coolant Temp)
  Constant5/1 -> Load Thermal Model/3(Air Temp)
  Battery Thermal Model/1(T_Batt) -> Tbatt/1
  Load Thermal Model/1(T_gen) -> TLoad/1
  Generator 3 Thermal Model/1(T_gen) -> Mux/3, Tgen3/1
  Mux/1 -> To Workspace6/1
  Gain/1 -> Demux/1

== system Boeing787_NewMission_ElectricalThermal_2013/Electrical/Transformer-rectifier ==
  vqd0 : Inport
  iDC : Inport  Port=2
  Constant1 : Constant  Value=270
  Constant2 : Constant  Value=1.0
  Control : Subsystem
  Sum1 : Sum  Inputs=|++
  Three-phase Full Bridge Rectifier : Subsystem  AncestorBlock=PowerFlowLib/Energy & Power Systems/Electrical/Rectifiers/Three-phase Full Bridge1  mask(Single-phase full bridge rectifier.){C=100e-6, Rc=1}
      mask prompts: C "Output capacitance (F):"; Rc "Circuit parasitic resistance (ohm):"
      mask help: Single-phase Full bridge rectifier. Lead resistance is added to make simulation possible.
  Transformer1 : Subsystem  AncestorBlock=PowerFlowLib/Energy & Power Systems/Electrical/Machines/Transformer  mask(Transformer){Rp=0.005, Rs=0.1, N1=400, N2=332*1.4}
      mask prompts: Rp "Primary Winding Resistance"; Rs "Secondary Winding Resistance"; N1 "Number of Turns in Primary"; N2 "Number of Turns in Secondary"
      mask help:
      | The user inputs and outputs are given below. Inputs to the model are:
      |
      | Block Inputs
      | #1: Primary voltage input [V]
      | #2: Secondary current input [A]
      |
      | Block Outputs
      | #1: Secondary voltage output [V]
      | #2: Primary current input [A]
      mask Help: eval('open(''Transformer Help.html'')');
      mask Display:
      | image(imread('Transformer.png'))
      | 
      | port_label('input',1,'{\bf V_i_n}','TexMode','on')
      | port_label('input',2,'{\bf I_o_u_t}','TexMode','on')
      | 
      | port_label('output',1,'{\bf V_o_u_t}','TexMode','on')
      | port_label('output',2,'{\bf I_i_n}','TexMode','on')
  vout : Outport
  iqd0 : Outport  Port=2
  wires:
  Transformer1/2(Iin) -> iqd0/1
  Transformer1/1(Vout) -> Three-phase Full Bridge Rectifier/2(vin)
  vqd0/1 -> Transformer1/1(Vin)
  Three-phase Full Bridge Rectifier/2(iin) -> Transformer1/2(Iout)
  iDC/1 -> Three-phase Full Bridge Rectifier/1(iout)
  Three-phase Full Bridge Rectifier/1(vout) -> Control/1(Vout), vout/1
  Constant1/1 -> Control/2(ref)
  Constant2/1 -> Sum1/1
  Control/1(u) -> Sum1/2
  Sum1/1 -> Three-phase Full Bridge Rectifier/3(u)

== system Boeing787_NewMission_ElectricalThermal_2013/Electrical/Transformer-rectifier1 ==
  vqd0 : Inport
  iDC : Inport  Port=2
  Constant : Constant
  Constant1 : Constant  Value=28
  Control : Subsystem
  Saturation : Saturate  UpperLimit=inf  LowerLimit=-inf
  Sum1 : Sum  Inputs=|++
  Three-phase Full Bridge1 : Subsystem  AncestorBlock=PowerFlowLib/Energy & Power Systems/Electrical/Rectifiers/Three-phase Full Bridge1  mask(Single-phase full bridge rectifier.){C=100e-6, Rc=1}
      mask prompts: C "Output capacitance (F):"; Rc "Circuit parasitic resistance (ohm):"
      mask help: Single-phase Full bridge rectifier. Lead resistance is added to make simulation possible.
  Transformer1 : Subsystem  AncestorBlock=PowerFlowLib/Energy & Power Systems/Electrical/Machines/Transformer  mask(Transformer){Rp=0.005, Rs=0.1, N1=400, N2=45}
      mask prompts: Rp "Primary Winding Resistance"; Rs "Secondary Winding Resistance"; N1 "Number of Turns in Primary"; N2 "Number of Turns in Secondary"
      mask help:
      | The user inputs and outputs are given below. Inputs to the model are:
      |
      | Block Inputs
      | #1: Primary voltage input [V]
      | #2: Secondary current input [A]
      |
      | Block Outputs
      | #1: Secondary voltage output [V]
      | #2: Primary current input [A]
      mask Help: eval('open(''Transformer Help.html'')');
      mask Display:
      | image(imread('Transformer.png'))
      | 
      | port_label('input',1,'{\bf V_i_n}','TexMode','on')
      | port_label('input',2,'{\bf I_o_u_t}','TexMode','on')
      | 
      | port_label('output',1,'{\bf V_o_u_t}','TexMode','on')
      | port_label('output',2,'{\bf I_i_n}','TexMode','on')
  vout : Outport
  iqd0 : Outport  Port=2
  wires:
  Three-phase Full Bridge1/1(vout) -> Control/1(Vout), vout/1
  iDC/1 -> Three-phase Full Bridge1/1(iout)
  Three-phase Full Bridge1/2(iin) -> Transformer1/2(Iout)
  vqd0/1 -> Transformer1/1(Vin)
  Transformer1/1(Vout) -> Three-phase Full Bridge1/2(vin)
  Transformer1/2(Iin) -> iqd0/1
  Constant1/1 -> Control/2(ref)
  Constant/1 -> Sum1/1
  Control/1(u) -> Sum1/2
  Sum1/1 -> Saturation/1
  Saturation/1 -> Three-phase Full Bridge1/3(u)

== system Boeing787_NewMission_ElectricalThermal_2013/Eng1/Gearbox ==
  w_engine : Inport
  T_gen : Inport  Port=2
  1-tran_efficiency : Gain  Gain=1-Gear_Efficiency/100  SaturateOnIntegerOverflow=on  OutDataTypeStr=Inherit: Same as input  ParamDataTypeStr=Inherit: Same as input
  Gain : Gain  Gain=Gear_Ratio
  Gain1 : Gain  Gain=Gear_Ratio
  Memory1 : Memory
  Sum : Sum  Inputs=-++  SaturateOnIntegerOverflow=on  InputSameDT=on  OutDataTypeStr=Inherit: Same as first input
  gear1 NL loss : Lookup  InputValues=[0;1000;2000;3000;4000;5000;6000]*2*pi/60  Table=[0;0.735;1.334;1.491;1.525;1.212;1.276]  SaturateOnIntegerOverflow=on
  tran_efficiency : Gain  Gain=Gear_Efficiency/4/100  SaturateOnIntegerOverflow=on  OutDataTypeStr=Inherit: Same as input  ParamDataTypeStr=Inherit: Same as input
  w_shaft : Outport
  T_shaft : Outport  Port=2
  wires:
  Gain/1 -> w_shaft/1
  Gain1/1 -> Memory1/1
  T_gen/1 -> Gain1/1, 1-tran_efficiency/1
  w_engine/1 -> Gain/1, gear1 NL loss/1
  gear1 NL loss/1 -> tran_efficiency/1
  Memory1/1 -> Sum/3
  1-tran_efficiency/1 -> Sum/2
  tran_efficiency/1 -> Sum/1
  Sum/1 -> T_shaft/1

== system Boeing787_NewMission_ElectricalThermal_2013/Eng1/Unit Conversion  ==
  Signal_in : Inport
  conv_fcn : Fcn  Expr=u(1)/745.69987
  Converted Signal Out : Outport
  wires:
  Signal_in/1 -> conv_fcn/1
  conv_fcn/1 -> Converted Signal Out/1

== system Boeing787_NewMission_ElectricalThermal_2013/Eng1/Unit Conversion 1 ==
  Signal_in : Inport
  conv_fcn : Fcn  Expr=u(1)/1.8
  Converted Signal Out : Outport
  wires:
  conv_fcn/1 -> Converted Signal Out/1
  Signal_in/1 -> conv_fcn/1

== system Boeing787_NewMission_ElectricalThermal_2013/Eng1/Unit Conversion 4 ==
  Signal_in : Inport
  conv_fcn : Fcn  Expr=u(1)/(1.450377e-1)
  Converted Signal Out : Outport
  wires:
  Signal_in/1 -> conv_fcn/1
  conv_fcn/1 -> Converted Signal Out/1

== system Boeing787_NewMission_ElectricalThermal_2013/Eng1/Unit Conversion 5 ==
  Signal_in : Inport
  conv_fcn : Fcn  Expr=u(1)*.45359237
  Converted Signal Out : Outport
  wires:
  Signal_in/1 -> conv_fcn/1
  conv_fcn/1 -> Converted Signal Out/1
